simulink model "BLDCmotor_FOC_R2017b_fixdt"  (R2025a)
settings: Solver=FixedStepDiscrete  StartTime=0  StopTime=0.5  FixedStep=Ts  MaxStep=1e-6  RelTol=1e-6  AbsTol=1e-6  EnableMultiTasking=on
PreLoadFcn:
  | addpath(pwd);
  | addpath(genpath('01_Libraries'));
  | addpath(genpath('02_Figures'));
  | addpath(genpath('03_CreateParamTable'));
InitFcn:
  | init_model;
values from neighbouring files (symbols this model uses):
  a_cpr = 65535    [init_model.m]
  a_elecAngle = 60    [init_model.m]
  a_elecoffset = a_elecPeriod/12    (= 30)    [init_model.m]
  a_elecPeriod = 360    [init_model.m]
  a_fcpr = 1/65535    (= 1.52590218967e-05)    [init_model.m]
  a_mechoffset = a_elecoffset/n_polePairs    (= 5)    [init_model.m]
  a_phaAdvMax = 25    [init_model.m]
  b_angleMeasEna = 1    [init_model.m]
  b_cruiseCtrlEna = 0    [init_model.m]
  b_diagEna = 0    [init_model.m]
  b_fieldWeakEna = 0    [init_model.m]
  cf_currFilt = 0.692    [init_model.m]
  cf_idKi = Ki / (f_ctrl)    (= 0.00409061543436)    [init_model.m]
  cf_idKp = Kp    (= 0.0523598775598)    [init_model.m]
  cf_iqKi = Ki / (f_ctrl)    (= 0.00409061543436)    [init_model.m]
  cf_iqKiLimProt = 60 / (f_ctrl)    (= 0.00375)    [init_model.m]
  cf_iqKp = Kp    (= 0.0523598775598)    [init_model.m]
  cf_KbLimProt = Simulink.Parameter    [init_model.m]
  cf_nKi = 20.4 / (f_ctrl)    (= 0.001275)    [init_model.m]
  cf_nKiLimProt = 20 / (f_ctrl)    (= 0.00125)    [init_model.m]
  cf_nKp = 1.18    [init_model.m]
  cf_speedCoef = round(f_ctrl * a_mechAngle * (pi/180) * (30/pi))    [init_model.m]
  CTRL_FOC = 2    [init_model.m]
  CTRL_SIN = 1    [init_model.m]
  dV_openRate = 1000 / (f_ctrl)    (= 0.0625)    [init_model.m]
  dz_cntTrnsDetHi = 40    [init_model.m]
  dz_cntTrnsDetLo = 20    [init_model.m]
  ff_gain = ((r_motn / i_sca) * ((GD32_Vd_max_margin) / v_bus))    (= 0.338958333333)    [init_model.m]
  GD32_Vd_max_margin = GD32_Vd_max - V_margin    (= 1627)    [init_model.m]
  GD32_Vq_max_M1 = sqrt(GD32_Vd_max_margin^2 - GD32_Vq_max_XA.^2)    [init_model.m]
  i_max = i_max * i_sca    (= 500)    [init_model.m]
  id_fieldWeakMax = 5 * i_sca    (= 250)    [init_model.m]
  iq_maxSca_M1 = sqrt(1 - iq_maxSca_XA.^2)    [init_model.m]
  mcu_model = GD32F103    (= 1)    [init_model.m]
  n_commAcvLo = 15    [init_model.m]
  n_commDeacvHi = 30    [init_model.m]
  n_cruiseMotTgt = 0    [init_model.m]
  n_fieldWeakAuthHi = 300    [init_model.m]
  n_fieldWeakAuthLo = 100    [init_model.m]
  n_max = 1950    [init_model.m]
  n_polePairs = 6    [init_model.m]
  n_stdStillDet = 3    [init_model.m]
  OPEN_MODE = 0    [init_model.m]
  r_cos_M1 = cos((a_elecAngle_XA + a_elecPeriod/12)*(pi/180))    [init_model.m]
  r_errInpTgtThres = 600    [init_model.m]
  r_fieldWeakHi = 1000    [init_model.m]
  r_fieldWeakLo = 750    [init_model.m]
  r_motn = r_mot/2    (= 0.25)    [init_model.m]
  r_sin3PhaA_M1 = sin3Arm + A*r_sinPhaA_M1    [init_model.m]
  r_sin3PhaB_M1 = sin3Arm + A*r_sinPhaB_M1    [init_model.m]
  r_sin3PhaC_M1 = sin3Arm + A*r_sinPhaC_M1    [init_model.m]
  r_sin_M1 = sin((a_elecAngle_XA + a_elecPeriod/12)*(pi/180))    [init_model.m]
  SPD_MODE = 2    [init_model.m]
  STM32_Vd_max_margin = STM32_Vd_max - V_margin    (= 940)    [init_model.m]
  STM32_Vq_max_M1 = sqrt(STM32_Vd_max_margin^2 - STM32_Vq_max_XA.^2)    [init_model.m]
  t_errDequal = 1.80 * f_ctrl    (= 28800)    [init_model.m]
  t_errQual = 0.24 * f_ctrl    (= 3840)    [init_model.m]
  tgt_scale = 2047    [init_model.m]
  TRQ_MODE = 3    [init_model.m]
  Ts = 5e-6    (= 5e-06)    [init_model.m]
  Ts_ctrl = 6e-5    (= 6e-05)    [init_model.m]
  v_bus = 24    [init_model.m]
  vec_hallToPos = [0 2 0 1 4 3 5 0]    [init_model.m]
  VLT_MODE = 1    [init_model.m]
  z_commutMap_M1 = [-1 -1  0  1  1  0 ... (first row only)    [init_model.m]
  z_ctrlModReq = TRQ_MODE    (= 3)    [init_model.m]
  z_ctrlTypSel = CTRL_FOC    (= 2)    [init_model.m]
  z_maxCntRst = 2000    [init_model.m]
  z_selPhaCurMeasABC = 2    [init_model.m]
undefined symbols (not defined in the file or in its folder): BLDCmotor_FOC_R2017b_fixdt, DiscIntNeverNeededParam, DWORK0, DWORK1, DWORK2, DWORK3, powergui, spspowerguiLib
libraries: BLDC_controller_Lib x18, simulink x13, prociolib x6, eePwmGenerator x6, eePwmGeneratorMultilevel x3, mcbpositiondecoderlib x2, slpidlib x2, spsControlledVoltageSourceLib x1, spsMultimeterLib x1, spsPermanentMagnetSynchronousMachineLib x1, spsUniversalBridgeLib x1, spsVoltageMeasurementLib x1
(part 4 of 6)

== system BLDCmotor_FOC_R2017b_fixdt/BLDC_controller/F05_Field_Oriented_Control/Clarke_Park_Transform_Forward ==
  note: Start filtering only when motor is enabled (circuit closed).
  b_motEna : Inport
  a_elecAngle : Inport  Port=2
  i_phaAB : Inport  Port=3
  i_phaBC : Inport  Port=4
  Action Port : ActionPort  ActionPortLabel=if(u1 == CTRL_FOC)
  Clarke_Transform : Subsystem
  Current_Filtering : Subsystem
  If2 : If  IfExpression=u1 ~= 0  ShowElse=off
  Park_Transform : Subsystem
  Scope : Scope  NumInputPorts=8
      settings: ActiveDisplayYMinimum=-1177.3322840678534  ActiveDisplayYMaximum=1058.8681928463843  DataLoggingVariableName=ScopeData4
  Sine_Cosine_Approximation : Subsystem
  r_sin : Outport  OutputWhenDisabled=reset  InitialOutput=0  VectorParamsAs1DForOutWhenUnconnected=off
  r_cos : Outport  Port=2  OutputWhenDisabled=reset  InitialOutput=0  VectorParamsAs1DForOutWhenUnconnected=off
  iq : Outport  Port=3  OutputWhenDisabled=reset  InitialOutput=0  VectorParamsAs1DForOutWhenUnconnected=off
  id : Outport  Port=4  OutputWhenDisabled=reset  InitialOutput=0  VectorParamsAs1DForOutWhenUnconnected=off
  iqAbs : Outport  Port=5  OutputWhenDisabled=reset  InitialOutput=0  VectorParamsAs1DForOutWhenUnconnected=off
  wires:
  [a_elecAngle] -> Sine_Cosine_Approximation/1(a_elecAngle)
  Sine_Cosine_Approximation/1(r_sin) -> [r_sin]
  Sine_Cosine_Approximation/2(r_cos) -> [r_cos]
  [b_motEna] -> If2/1
  If2/1 -> Current_Filtering/Action
  Current_Filtering/2(iqAbs) -> [iqAbs]
  [i_phaAB] -> Clarke_Transform/1(i_phaAB)
  [i_phaBC] -> Clarke_Transform/2(i_phaBC)
  Current_Filtering/3(id) -> Scope/4, [id]
  Park_Transform/1(iq_Raw) -> Scope/2, Current_Filtering/1(iq_raw)
  Current_Filtering/1(iq) -> Scope/1, [iq]
  Park_Transform/2(id_Raw) -> Scope/3, Current_Filtering/2(id_raw)
  Clarke_Transform/2(i_beta) -> Scope/6, Park_Transform/2(i_beta)
  [r_cos] -> Scope/8, Park_Transform/4(r_cos)
  [r_sin] -> Scope/7, Park_Transform/3(r_sin)
  Clarke_Transform/1(i_alpha) -> Scope/5, Park_Transform/1(i_apha)
  b_motEna/1 -> [b_motEna]
  i_phaAB/1 -> [i_phaAB]
  i_phaBC/1 -> [i_phaBC]
  a_elecAngle/1 -> [a_elecAngle]
  [id] -> id/1
  [iq] -> iq/1
  [iqAbs] -> iqAbs/1
  [r_cos] -> r_cos/1
  [r_sin] -> r_sin/1

== system BLDCmotor_FOC_R2017b_fixdt/BLDC_controller/F05_Field_Oriented_Control/Clarke_Park_Transform_Inverse ==
  Vq : Inport
  Vd : Inport  Port=2
  r_sin : Inport  Port=3
  r_cos : Inport  Port=4
  Action Port : ActionPort  ActionPortLabel=if(u1 == CTRL_FOC)
  Inv_Clarke_Transform : Subsystem
  Inv_Park_Transform : Subsystem
  Scope : Scope  NumInputPorts=5
      settings: ActiveDisplayYMinimum=-2289.157291869059  ActiveDisplayYMaximum=2435.0032996145992  DataLoggingVariableName=ScopeData3
  V_phaABC_FOC : Outport  OutputWhenDisabled=reset  InitialOutput=0  VectorParamsAs1DForOutWhenUnconnected=off
  wires:
  [V_phaABC_FOC] -> V_phaABC_FOC/1
  Vd/1 -> [Vd]
  r_cos/1 -> [r_cos]
  r_sin/1 -> [r_sin]
  Vq/1 -> [Vq]
  Inv_Clarke_Transform/1(V_phaABC_FOC) -> Scope/5, [V_phaABC_FOC]
  [r_cos] -> Inv_Park_Transform/4(r_cos)
  [Vq] -> Scope/3, Inv_Park_Transform/1(Vq)
  Inv_Park_Transform/1(V_alpha) -> Scope/1, Inv_Clarke_Transform/1(V_alpha)
  Inv_Park_Transform/2(V_beta) -> Scope/4, Inv_Clarke_Transform/2(V_beta)
  [r_sin] -> Inv_Park_Transform/3(r_sin)
  [Vd] -> Scope/2, Inv_Park_Transform/2(Vd)

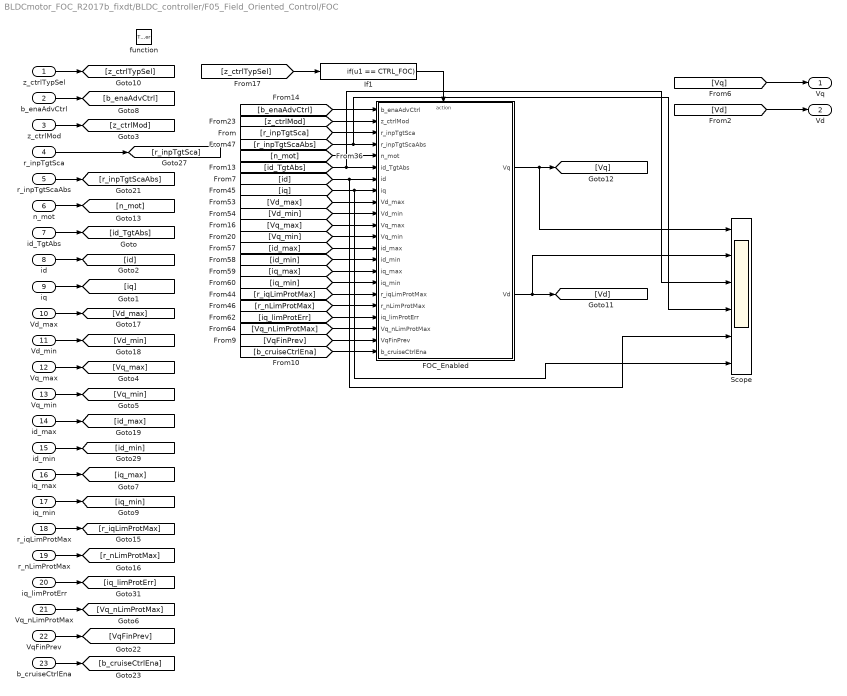
== system BLDCmotor_FOC_R2017b_fixdt/BLDC_controller/F05_Field_Oriented_Control/FOC ==
  z_ctrlTypSel : Inport
  b_enaAdvCtrl : Inport  Port=2
  z_ctrlMod : Inport  Port=3
  r_inpTgtSca : Inport  Port=4
  r_inpTgtScaAbs : Inport  Port=5
  n_mot : Inport  Port=6
  id_TgtAbs : Inport  Port=7
  id : Inport  Port=8
  iq : Inport  Port=9
  Vd_max : Inport  Port=10
  Vd_min : Inport  Port=11
  Vq_max : Inport  Port=12
  Vq_min : Inport  Port=13
  id_max : Inport  Port=14
  id_min : Inport  Port=15
  iq_max : Inport  Port=16
  iq_min : Inport  Port=17
  r_iqLimProtMax : Inport  Port=18
  r_nLimProtMax : Inport  Port=19
  iq_limProtErr : Inport  Port=20
  Vq_nLimProtMax : Inport  Port=21
  VqFinPrev : Inport  Port=22
  b_cruiseCtrlEna : Inport  Port=23
  function : TriggerPort  TriggerType=function-call  VariantControl=Variant
  FOC_Enabled : Subsystem
  If1 : If  IfExpression=u1 == CTRL_FOC  ShowElse=off
  Scope : Scope  NumInputPorts=6
      settings: ActiveDisplayYMinimum=-3867.0934008019167  ActiveDisplayYMaximum=2204.1532756193237  DataLoggingVariableName=ScopeData7
  Vq : Outport  VectorParamsAs1DForOutWhenUnconnected=off
  Vd : Outport  Port=2  VectorParamsAs1DForOutWhenUnconnected=off
  wires:
  [Vq] -> Vq/1
  [Vd] -> Vd/1
  r_inpTgtSca/1 -> [r_inpTgtSca]
  z_ctrlMod/1 -> [z_ctrlMod]
  b_enaAdvCtrl/1 -> [b_enaAdvCtrl]
  iq/1 -> [iq]
  id_min/1 -> [id_min]
  id_max/1 -> [id_max]
  Vd_max/1 -> [Vd_max]
  id_TgtAbs/1 -> [id_TgtAbs]
  id/1 -> [id]
  Vd_min/1 -> [Vd_min]
  Vq_min/1 -> [Vq_min]
  Vq_max/1 -> [Vq_max]
  Vq_nLimProtMax/1 -> [Vq_nLimProtMax]
  iq_limProtErr/1 -> [iq_limProtErr]
  iq_min/1 -> [iq_min]
  iq_max/1 -> [iq_max]
  n_mot/1 -> [n_mot]
  r_iqLimProtMax/1 -> [r_iqLimProtMax]
  r_nLimProtMax/1 -> [r_nLimProtMax]
  r_inpTgtScaAbs/1 -> [r_inpTgtScaAbs]
  VqFinPrev/1 -> [VqFinPrev]
  b_cruiseCtrlEna/1 -> [b_cruiseCtrlEna]
  [b_cruiseCtrlEna] -> FOC_Enabled/22(b_cruiseCtrlEna)
  [r_nLimProtMax] -> FOC_Enabled/18(r_nLimProtMax)
  [r_inpTgtSca] -> FOC_Enabled/3(r_inpTgtSca)
  [r_inpTgtScaAbs] -> Scope/4, FOC_Enabled/4(r_inpTgtScaAbs)
  [Vd_max] -> FOC_Enabled/9(Vd_max)
  [b_enaAdvCtrl] -> FOC_Enabled/1(b_enaAdvCtrl)
  [r_iqLimProtMax] -> FOC_Enabled/17(r_iqLimProtMax)
  [iq_min] -> FOC_Enabled/16(iq_min)
  [iq] -> Scope/6, FOC_Enabled/8(iq)
  [z_ctrlMod] -> FOC_Enabled/2(z_ctrlMod)
  [n_mot] -> FOC_Enabled/5(n_mot)
  [Vq_min] -> FOC_Enabled/12(Vq_min)
  [Vq_nLimProtMax] -> FOC_Enabled/20(Vq_nLimProtMax)
  [id_TgtAbs] -> Scope/3, FOC_Enabled/6(id_TgtAbs)
  [id_max] -> FOC_Enabled/13(id_max)
  [iq_max] -> FOC_Enabled/15(iq_max)
  [Vd_min] -> FOC_Enabled/10(Vd_min)
  [id] -> Scope/5, FOC_Enabled/7(id)
  [VqFinPrev] -> FOC_Enabled/21(VqFinPrev)
  [id_min] -> FOC_Enabled/14(id_min)
  [Vq_max] -> FOC_Enabled/11(Vq_max)
  [iq_limProtErr] -> FOC_Enabled/19(iq_limProtErr)
  [z_ctrlTypSel] -> If1/1
  If1/1 -> FOC_Enabled/Action
  z_ctrlTypSel/1 -> [z_ctrlTypSel]
  FOC_Enabled/1(Vq) -> Scope/1, [Vq]
  FOC_Enabled/2(Vd) -> Scope/2, [Vd]

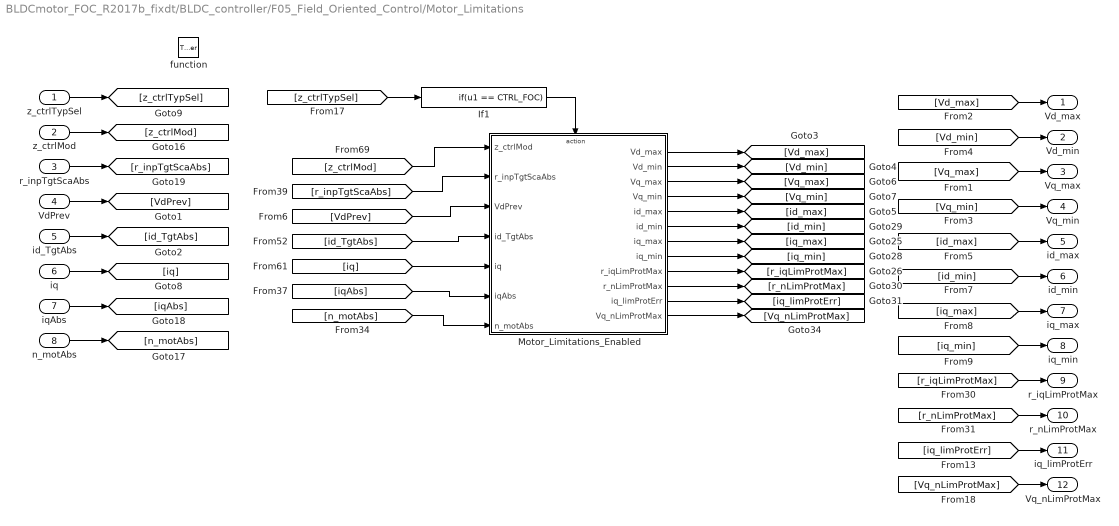
== system BLDCmotor_FOC_R2017b_fixdt/BLDC_controller/F05_Field_Oriented_Control/Motor_Limitations ==
  z_ctrlTypSel : Inport
  z_ctrlMod : Inport  Port=2
  r_inpTgtScaAbs : Inport  Port=3
  VdPrev : Inport  Port=4
  id_TgtAbs : Inport  Port=5
  iq : Inport  Port=6
  iqAbs : Inport  Port=7
  n_motAbs : Inport  Port=8
  function : TriggerPort  TriggerType=function-call  VariantControl=Variant
  If1 : If  IfExpression=u1 == CTRL_FOC  ShowElse=off
  Motor_Limitations_Enabled : Subsystem
  Vd_max : Outport  VectorParamsAs1DForOutWhenUnconnected=off
  Vd_min : Outport  Port=2  VectorParamsAs1DForOutWhenUnconnected=off
  Vq_max : Outport  Port=3  VectorParamsAs1DForOutWhenUnconnected=off
  Vq_min : Outport  Port=4  VectorParamsAs1DForOutWhenUnconnected=off
  id_max : Outport  Port=5  VectorParamsAs1DForOutWhenUnconnected=off
  id_min : Outport  Port=6  VectorParamsAs1DForOutWhenUnconnected=off
  iq_max : Outport  Port=7  VectorParamsAs1DForOutWhenUnconnected=off
  iq_min : Outport  Port=8  VectorParamsAs1DForOutWhenUnconnected=off
  r_iqLimProtMax : Outport  Port=9  VectorParamsAs1DForOutWhenUnconnected=off
  r_nLimProtMax : Outport  Port=10  VectorParamsAs1DForOutWhenUnconnected=off
  iq_limProtErr : Outport  Port=11  VectorParamsAs1DForOutWhenUnconnected=off
  Vq_nLimProtMax : Outport  Port=12  VectorParamsAs1DForOutWhenUnconnected=off
  wires:
  [Vq_min] -> Vq_min/1
  [Vq_max] -> Vq_max/1
  VdPrev/1 -> [VdPrev]
  id_TgtAbs/1 -> [id_TgtAbs]
  [Vd_max] -> Vd_max/1
  [Vd_min] -> Vd_min/1
  [id_min] -> id_min/1
  [id_max] -> id_max/1
  [iq_max] -> iq_max/1
  [iq_min] -> iq_min/1
  iq/1 -> [iq]
  [iq_limProtErr] -> iq_limProtErr/1
  [Vq_nLimProtMax] -> Vq_nLimProtMax/1
  z_ctrlMod/1 -> [z_ctrlMod]
  n_motAbs/1 -> [n_motAbs]
  iqAbs/1 -> [iqAbs]
  r_inpTgtScaAbs/1 -> [r_inpTgtScaAbs]
  [r_nLimProtMax] -> r_nLimProtMax/1
  [r_iqLimProtMax] -> r_iqLimProtMax/1
  [z_ctrlMod] -> Motor_Limitations_Enabled/1(z_ctrlMod)
  [r_inpTgtScaAbs] -> Motor_Limitations_Enabled/2(r_inpTgtScaAbs)
  [VdPrev] -> Motor_Limitations_Enabled/3(VdPrev)
  [id_TgtAbs] -> Motor_Limitations_Enabled/4(id_TgtAbs)
  [iq] -> Motor_Limitations_Enabled/5(iq)
  [iqAbs] -> Motor_Limitations_Enabled/6(iqAbs)
  [n_motAbs] -> Motor_Limitations_Enabled/7(n_motAbs)
  Motor_Limitations_Enabled/1(Vd_max) -> [Vd_max]
  Motor_Limitations_Enabled/2(Vd_min) -> [Vd_min]
  Motor_Limitations_Enabled/3(Vq_max) -> [Vq_max]
  Motor_Limitations_Enabled/4(Vq_min) -> [Vq_min]
  Motor_Limitations_Enabled/5(id_max) -> [id_max]
  Motor_Limitations_Enabled/6(id_min) -> [id_min]
  Motor_Limitations_Enabled/7(iq_max) -> [iq_max]
  Motor_Limitations_Enabled/8(iq_min) -> [iq_min]
  Motor_Limitations_Enabled/9(r_iqLimProtMax) -> [r_iqLimProtMax]
  Motor_Limitations_Enabled/10(r_nLimProtMax) -> [r_nLimProtMax]
  Motor_Limitations_Enabled/11(iq_limProtErr) -> [iq_limProtErr]
  Motor_Limitations_Enabled/12(Vq_nLimProtMax) -> [Vq_nLimProtMax]
  [z_ctrlTypSel] -> If1/1
  If1/1 -> Motor_Limitations_Enabled/Action
  z_ctrlTypSel/1 -> [z_ctrlTypSel]

== system BLDCmotor_FOC_R2017b_fixdt/BLDC_controller/F06_Control_Type_Management/COM_Method ==
  VqFin : Inport
  z_pos : Inport  Port=2
  Action Port : ActionPort  ActionPortLabel=else
  Divide2 : Product  Inputs=**  RndMeth=Simplest  OutDataTypeStr=Inherit: Same as first input
  z_commutMap_M1 : LookupNDDirect  InputsSelectThisObjectFromTable=Vector  Table=z_commutMap_M1  DiagnosticForOutOfRangeInput=None  TableDataTypeStr=int8
  V_phaABC_COM : Outport  VectorParamsAs1DForOutWhenUnconnected=off
  wires:
  Divide2/1 -> [V_phaABC_COM]
  [z_pos] -> z_commutMap_M1/1
  z_commutMap_M1/1 -> Divide2/2
  [VqFin] -> Divide2/1
  VqFin/1 -> [VqFin]
  z_pos/1 -> [z_pos]
  [V_phaABC_COM] -> V_phaABC_COM/1

== system BLDCmotor_FOC_R2017b_fixdt/BLDC_controller/F06_Control_Type_Management/FOC_Method ==
  V_phaABC_FOC_in : Inport
  Action Port : ActionPort  ActionPortLabel=if(u1 ~= 0)
  V_phaABC_FOC : Outport  VectorParamsAs1DForOutWhenUnconnected=off
  wires:
  V_phaABC_FOC_in/1 -> V_phaABC_FOC/1

== system BLDCmotor_FOC_R2017b_fixdt/BLDC_controller/F06_Control_Type_Management/SIN_Method ==
  note: Sinusoidal With 3rd Harmonic
  VqFin : Inport
  a_elecAngle : Inport  Port=2
  z_dir : Inport  Port=3
  r_fieldWeak : Inport  Port=4
  Action Port : ActionPort  ActionPortLabel=elseif(u2 ~= 0)
  Constant : Constant  Value=0  OutDataTypeStr=uint8
  Divide2 : Product  Inputs=**  RndMeth=Simplest  OutDataTypeStr=Inherit: Same as first input
  Final_Phase_Advance_Calculation : Subsystem
  Mux2 : Mux  Inputs=3
  a_elecAngle_XA : PreLookup  BreakpointsData=a_elecAngle_XA  OutputSelection=Index only  IndexSearchMethod=Evenly spaced points  BeginIndexSearchUsingPreviousIndexResult=on  IndexDataTypeStr=uint8  RndMeth=Simplest
  r_sin3PhaA_M1 : Interpolation_n-D  NumberOfTableDimensions=1  Table=r_sin3PhaA_M1  InterpMethod=Flat  ExtrapMethod=Clip  RemoveProtectionIndex=on  ValidIndexMayReachLast=on  OutDataTypeStr=fixdt(1,16,14)  InternalRulePriority=Speed  RndMeth=Simplest
      settings: InputPortMap=u0,u1
  r_sin3PhaB_M1 : Interpolation_n-D  NumberOfTableDimensions=1  Table=r_sin3PhaB_M1  InterpMethod=Flat  ExtrapMethod=Clip  RemoveProtectionIndex=on  ValidIndexMayReachLast=on  OutDataTypeStr=fixdt(1,16,14)  InternalRulePriority=Speed  RndMeth=Simplest
      settings: InputPortMap=u0,u1
  r_sin3PhaC_M1 : Interpolation_n-D  NumberOfTableDimensions=1  Table=r_sin3PhaC_M1  InterpMethod=Flat  ExtrapMethod=Clip  RemoveProtectionIndex=on  ValidIndexMayReachLast=on  OutDataTypeStr=fixdt(1,16,14)  InternalRulePriority=Speed  RndMeth=Simplest
      settings: InputPortMap=u0,u1
  V_phaABC_SIN : Outport  VectorParamsAs1DForOutWhenUnconnected=off
  wires:
  a_elecAngle_XA/1 -> r_sin3PhaC_M1/1, r_sin3PhaB_M1/1, r_sin3PhaA_M1/1
  Constant/1 -> r_sin3PhaC_M1/2, r_sin3PhaB_M1/2, r_sin3PhaA_M1/2
  Final_Phase_Advance_Calculation/1(a_elecAngleAdv) -> a_elecAngle_XA/1
  a_elecAngle/1 -> [a_elecAngle]
  r_fieldWeak/1 -> [r_fieldWeak]
  z_dir/1 -> [z_dir]
  VqFin/1 -> [VqFin]
  [a_elecAngle] -> Final_Phase_Advance_Calculation/1(a_elecAngle)
  [z_dir] -> Final_Phase_Advance_Calculation/2(z_dir)
  [r_fieldWeak] -> Final_Phase_Advance_Calculation/3(r_fieldWeak)
  [V_phaABC_SIN] -> V_phaABC_SIN/1
  [VqFin] -> Divide2/1
  r_sin3PhaA_M1/1 -> Mux2/1
  r_sin3PhaB_M1/1 -> Mux2/2
  r_sin3PhaC_M1/1 -> Mux2/3
  Mux2/1 -> Divide2/2
  Divide2/1 -> [V_phaABC_SIN]

== system BLDCmotor_FOC_R2017b_fixdt/BLDC_model_open1/powergui/EquivalentModel1 ==
  Gates : Subsystem
  Sources : Subsystem
  State-Space : S-Function  FunctionName=sfun_spssw_discc  Parameters=S.Ts,S.A, S.B, S.C, S.D, S.x0, S.EnableUseOfTLC,S.SwitchResistance ,S.SwitchType, S.SwitchGateInitialValue, S.OutputsToResetToZero, S.TBEON,S.SaveMatrices,S.BufferSize  SFunctionDeploymentMode=off  EnableBusSupport=off
  Status : Subsystem
  Yout : Subsystem
  wires:
  State-Space/1 -> Yout/1(v,i)
  State-Space/2 -> Status/1(status)
  Sources/1(u) -> State-Space/1
  Gates/1(gates) -> State-Space/2

== system BLDCmotor_FOC_R2017b_fixdt/PWM_gates/MCU_VD_Selector/Default_Control_Type ==
  1 : Inport
  Action Port : ActionPort
  2 : Outport  VectorParamsAs1DForOutWhenUnconnected=off
  wires:
  1/1 -> 2/1

== system BLDCmotor_FOC_R2017b_fixdt/PWM_gates/MCU_VD_Selector/Default_Control_Type1 ==
  1 : Inport
  Action Port : ActionPort
  2 : Outport  VectorParamsAs1DForOutWhenUnconnected=off
  wires:
  1/1 -> 2/1

== system BLDCmotor_FOC_R2017b_fixdt/PWM_gates/PWM_generator1/__InputSSForSFun__ ==
  DC : Inport  SampleTime=Ts
  __UniqueOutportName__1__ : Outport  VectorParamsAs1DForOutWhenUnconnected=off
  wires:
  DC/1 -> __UniqueOutportName__1__/1

== system BLDCmotor_FOC_R2017b_fixdt/PWM_gates/PWM_generator1/__OutputSSForSFun__ ==
  __UniqueInportName__1__ : Inport
  PWM : Outport  VectorParamsAs1DForOutWhenUnconnected=off
  wires:
  __UniqueInportName__1__/1 -> PWM/1

== system BLDCmotor_FOC_R2017b_fixdt/PWM_gates/PWM_generator12/__InputSSForSFun__ ==
  DC : Inport  SampleTime=Ts
  __UniqueOutportName__1__ : Outport  VectorParamsAs1DForOutWhenUnconnected=off
  wires:
  DC/1 -> __UniqueOutportName__1__/1

== system BLDCmotor_FOC_R2017b_fixdt/PWM_gates/PWM_generator12/__OutputSSForSFun__ ==
  __UniqueInportName__1__ : Inport
  PWM : Outport  VectorParamsAs1DForOutWhenUnconnected=off
  wires:
  __UniqueInportName__1__/1 -> PWM/1

== system BLDCmotor_FOC_R2017b_fixdt/PWM_gates/PWM_generator2/__InputSSForSFun__ ==
  DC : Inport  SampleTime=Ts
  __UniqueOutportName__1__ : Outport  VectorParamsAs1DForOutWhenUnconnected=off
  wires:
  DC/1 -> __UniqueOutportName__1__/1

== system BLDCmotor_FOC_R2017b_fixdt/PWM_gates/PWM_generator2/__OutputSSForSFun__ ==
  __UniqueInportName__1__ : Inport
  PWM : Outport  VectorParamsAs1DForOutWhenUnconnected=off
  wires:
  __UniqueInportName__1__/1 -> PWM/1

== system BLDCmotor_FOC_R2017b_fixdt/PWM_gates/PWM_generator3/__InputSSForSFun__ ==
  DC : Inport  SampleTime=Ts
  __UniqueOutportName__1__ : Outport  VectorParamsAs1DForOutWhenUnconnected=off
  wires:
  DC/1 -> __UniqueOutportName__1__/1

== system BLDCmotor_FOC_R2017b_fixdt/PWM_gates/PWM_generator3/__OutputSSForSFun__ ==
  __UniqueInportName__1__ : Inport
  PWM : Outport  VectorParamsAs1DForOutWhenUnconnected=off
  wires:
  __UniqueInportName__1__/1 -> PWM/1

== system BLDCmotor_FOC_R2017b_fixdt/PWM_gates/PWM_generator4/__InputSSForSFun__ ==
  DC : Inport  SampleTime=Ts
  __UniqueOutportName__1__ : Outport  VectorParamsAs1DForOutWhenUnconnected=off
  wires:
  DC/1 -> __UniqueOutportName__1__/1

== system BLDCmotor_FOC_R2017b_fixdt/PWM_gates/PWM_generator4/__OutputSSForSFun__ ==
  __UniqueInportName__1__ : Inport
  PWM : Outport  VectorParamsAs1DForOutWhenUnconnected=off
  wires:
  __UniqueInportName__1__/1 -> PWM/1

== system BLDCmotor_FOC_R2017b_fixdt/PWM_gates/PWM_generator5/__InputSSForSFun__ ==
  DC : Inport  SampleTime=Ts
  __UniqueOutportName__1__ : Outport  VectorParamsAs1DForOutWhenUnconnected=off
  wires:
  DC/1 -> __UniqueOutportName__1__/1

== system BLDCmotor_FOC_R2017b_fixdt/PWM_gates/PWM_generator5/__OutputSSForSFun__ ==
  __UniqueInportName__1__ : Inport
  PWM : Outport  VectorParamsAs1DForOutWhenUnconnected=off
  wires:
  __UniqueInportName__1__/1 -> PWM/1

== system BLDCmotor_FOC_R2017b_fixdt/Power Stage/Variant Subsystem/GD32F103 ==
  Vd_max1 : Constant  Value=GD32_Vd_max_margin  OutDataTypeStr=fixdt(1,16,4)
  Vd_max_margin : Outport
  wires:
  Vd_max1/1 -> Vd_max_margin/1

== system BLDCmotor_FOC_R2017b_fixdt/Power Stage/Variant Subsystem/STM32F103 ==
  Vd_max3 : Constant  Value=STM32_Vd_max_margin  OutDataTypeStr=fixdt(1,16,4)
  Vd_max_margin : Outport
  wires:
  Vd_max3/1 -> Vd_max_margin/1

== system BLDCmotor_FOC_R2017b_fixdt/BLDC_controller/F01_Estimations/F01_04_Speed_Estimation/Raw_Motor_Speed_Estimation ==
  note: Speed calculations:
      | Speed_radps = (f_ctrl_Hz * Mechanical_angle_radps) / z_counter
      | cf_spd_coef = f_ctrl_Hz * Mechanical_angle_deg * pi/180 * 30/pi
      | Speed_radps = cf_spd_coef / z_counter
  note: Counter hold
  note: • In steady state, switch to 4 interval speed calculation for better accuracy.
      | • In transient, switch to 1 interval interval spped calculation for fast detection of the speed change.
  note: This switch is to manage when direction changes. In this case, the counter measures both the time to go and return (so twice the time) within the Hall change. However, the angle to stand-still is not known. As a work around just use the previous motor speed in absolute value.
  note: At stand-still the Hall sensor toggles if the motor is stoped at the edge of Hall change. This switch is to manage this situation and avoid unexpected behavior.
  z_dir : Inport
  z_dirPrev : Inport  Port=2
  z_counterRawPrev : Inport  Port=3
  n_motAbsPrev : Inport  Port=4
  Action Port : ActionPort  ActionPortLabel=if(u1 ~= 0)
  1-D Lookup Table : Lookup_n-D  Commented=on  NumberOfTableDimensions=1  BreakpointsForDimension1=1:8000  IndexSearchMethod=Evenly spaced points  BeginIndexSearchUsingPreviousIndexResult=on  Table=1 ./ (1:8000)  ExtrapMethod=Clip  RemoveProtectionInput=on  UseLastTableValue=on  ApplyFullPrecisionForLinearInterpolation=on  InternalRulePriority=Speed  OutDataTypeStr=fixdt(0,16,15)  RndMeth=Simplest
  Abs2 : Abs  OutDataTypeStr=Inherit: Inherit via back propagation  RndMeth=Zero  SaturateOnIntegerOverflow=off
  Constant4 : Constant  Value=0  OutDataTypeStr=Inherit: Inherit via back propagation
  Divide11 : Product  Inputs=**  RndMeth=Simplest  OutDataTypeStr=Inherit: Same as first input
  Divide13 : Product  Inputs=*/  OutDataTypeStr=fixdt(1,16,4)  RndMeth=Simplest
  Divide14 : Product  Inputs=*/  OutDataTypeStr=Inherit: Inherit via back propagation  RndMeth=Simplest
  From2 : From  Commented=on  GotoTag=cf_speedCoef
  From3 : From  Commented=on  GotoTag=z_counter
  Logical Operator1 : Logic  AllPortsSameDT=off  OutDataTypeStr=boolean
  Product : Product  Commented=on  OutDataTypeStr=int16  RndMeth=Simplest
  Relational Operator4 : RelationalOperator  Operator=~=  OutDataTypeStr=boolean  RndMeth=Simplest  InputSameDT=off
  Sum1 : Sum  Commented=on  Inputs=++++  InputSameDT=on  RndMeth=Simplest  OutDataTypeStr=Inherit: Same as first input
  Sum13 : Sum  Inputs=++++  InputSameDT=on  RndMeth=Simplest  OutDataTypeStr=Inherit: Same as first input
  Sum7 : Sum  Inputs=+-  InputSameDT=on  RndMeth=Simplest  OutDataTypeStr=Inherit: Same as first input
  Switch1 : Switch  Tag=struct('comment',struct('text','','placement',1),'logdata',struct('maxnumvals',inf,'plotchannels',[],'loggingmode',3,'channels',1),'output',struct('variable','','description','','name','$S_$B','width',1,'address','','max',NaN,'min',NaN,'class','default','type','CONTINUOUS','scaling','','lsb',1,'offset',0,'arb',0,'freeze',1,'unit','','autoscalingmode',1,'lowerheadroom',1,'upperheadroom',1,'headroomunit','bit','keepdatatype',1,'checkmin',0,'checkmax',0,'castoutput',0,'show',0),'threshold',struct('variable','','description','','name','$S_$B_threshold','width',1,'address','','max',NaN,'min',NaN,'class','default','type','CONTINUOUS','scaling','','lsb',1,'offset',0,'arb',0,'freeze',1,'unit','','keepdatatype',1,'value','0','scalar',0,'criteria',3),'scalingvalid',0,'date',733087.49614628474,'inheritscaling',0)  Criteria=u2 ~= 0  SaturateOnIntegerOverflow=off
      settings: AttributesFormatString=threshold=%<threshold>\nCriteria : %<Criteria>
  Switch2 : Switch  Tag=struct('comment',struct('text','','placement',1),'logdata',struct('maxnumvals',inf,'plotchannels',[],'loggingmode',3,'channels',1),'output',struct('variable','','description','','name','$S_$B','width',1,'address','','max',NaN,'min',NaN,'class','default','type','CONTINUOUS','scaling','','lsb',1,'offset',0,'arb',0,'freeze',1,'unit','','autoscalingmode',1,'lowerheadroom',1,'upperheadroom',1,'headroomunit','bit','keepdatatype',1,'checkmin',0,'checkmax',0,'castoutput',0,'show',0),'threshold',struct('variable','','description','','name','$S_$B_threshold','width',1,'address','','max',NaN,'min',NaN,'class','default','type','CONTINUOUS','scaling','','lsb',1,'offset',0,'arb',0,'freeze',1,'unit','','keepdatatype',1,'value','0','scalar',0,'criteria',3),'scalingvalid',0,'date',733087.49614628474,'inheritscaling',0)  Criteria=u2 ~= 0  SaturateOnIntegerOverflow=off
      settings: AttributesFormatString=threshold=%<threshold>\nCriteria : %<Criteria>
  Switch3 : Switch  Tag=struct('comment',struct('text','','placement',1),'logdata',struct('maxnumvals',inf,'plotchannels',[],'loggingmode',3,'channels',1),'output',struct('variable','','description','','name','$S_$B','width',1,'address','','max',NaN,'min',NaN,'class','default','type','CONTINUOUS','scaling','','lsb',1,'offset',0,'arb',0,'freeze',1,'unit','','autoscalingmode',1,'lowerheadroom',1,'upperheadroom',1,'headroomunit','bit','keepdatatype',1,'checkmin',0,'checkmax',0,'castoutput',0,'show',0),'threshold',struct('variable','','description','','name','$S_$B_threshold','width',1,'address','','max',NaN,'min',NaN,'class','default','type','CONTINUOUS','scaling','','lsb',1,'offset',0,'arb',0,'freeze',1,'unit','','keepdatatype',1,'value','0','scalar',0,'criteria',3),'scalingvalid',0,'date',733087.49614628474,'inheritscaling',0)  Criteria=u2 ~= 0  SaturateOnIntegerOverflow=off
      settings: AttributesFormatString=threshold=%<threshold>\nCriteria : %<Criteria>
  UnitDelay{1..5} (5 alike) : UnitDelay  SampleTime=-1  HasFrameUpgradeWarning=on
      settings: AttributesFormatString=Ini=%<X0>
  UnitDelay6 : UnitDelay  Commented=on  SampleTime=-1  HasFrameUpgradeWarning=on
      settings: AttributesFormatString=Ini=%<X0>
  UnitDelay7 : UnitDelay  Commented=on  SampleTime=-1  HasFrameUpgradeWarning=on
      settings: AttributesFormatString=Ini=%<X0>
  UnitDelay8 : UnitDelay  Commented=on  SampleTime=-1  HasFrameUpgradeWarning=on
      settings: AttributesFormatString=Ini=%<X0>
  cf_speedCoef : Constant  Value=cf_speedCoef  OutDataTypeStr=fixdt(0,16,0)
  dz_cntTrnsDet : Relay  OnSwitchValue=dz_cntTrnsDetHi  OffSwitchValue=dz_cntTrnsDetLo  OutDataTypeStr=boolean
  g_Ha : Gain  Commented=on  Gain=4  OutDataTypeStr=Inherit: Inherit via back propagation  RndMeth=Zero  ParamDataTypeStr=Inherit: Same as input
  z_counter : Outport  InitialOutput=z_maxCntRst  VectorParamsAs1DForOutWhenUnconnected=off
  dz_trnsDet : Outport  Port=2  VectorParamsAs1DForOutWhenUnconnected=off
  n_motRaw : Outport  Port=3  VectorParamsAs1DForOutWhenUnconnected=off
  wires:
  z_dir/1 -> [z_dir]
  z_dirPrev/1 -> [z_dirPrev]
  z_counterRawPrev/1 -> [z_counterRawPrev]
  [z_dir] -> Divide11/2
  UnitDelay3/1 -> UnitDelay2/1, Sum13/2
  UnitDelay5/1 -> UnitDelay3/1, Sum13/3
  [z_counter] -> UnitDelay5/1, Sum13/4
  Sum13/1 -> Divide13/2
  [z_counter] -> Divide14/2
  [cf_speedCoef] -> Divide14/1
  UnitDelay4/1 -> Sum7/2
  [z_counter] -> UnitDelay4/1, Sum7/1
  Sum7/1 -> Abs2/1
  Abs2/1 -> dz_cntTrnsDet/1
  cf_speedCoef/1 -> [cf_speedCoef]
  UnitDelay2/1 -> Sum13/1
  [z_dir] -> Relational Operator4/1
  [z_dirPrev] -> Relational Operator4/2
  UnitDelay1/1 -> Logical Operator1/2
  Relational Operator4/1 -> UnitDelay1/1, Switch2/2, Logical Operator1/1
  Logical Operator1/1 -> Switch3/2
  Switch2/1 -> Switch3/3
  Constant4/1 -> Switch3/1
  Switch3/1 -> Divide11/1
  n_motAbsPrev/1 -> [n_motAbsPrev]
  [n_motAbsPrev] -> Switch2/1
  [z_counterRawPrev] -> z_counter/1, [z_counter]
  dz_cntTrnsDet/1 -> [dz_trnsDet], dz_trnsDet/1
  Divide11/1 -> n_motRaw/1
  [dz_trnsDet] -> Switch1/2
  Switch1/1 -> Switch2/3
  Divide14/1 -> Switch1/1
  [cf_speedCoef] -> Divide13/1
  Divide13/1 -> Switch1/3
  UnitDelay8/1 -> UnitDelay7/1, Sum1/3
  Sum1/1 -> 1-D Lookup Table/1
  UnitDelay7/1 -> UnitDelay6/1, Sum1/2
  UnitDelay6/1 -> Sum1/1
  From3/1 -> UnitDelay8/1, Sum1/4
  1-D Lookup Table/1 -> Product/2
  From2/1 -> Product/1

== system BLDCmotor_FOC_R2017b_fixdt/BLDC_controller/F03_Control_Mode_Manager/F03_03_Input_Target_Synthesis/Default_Control_Type ==
  r_inpTgtConv : Inport
  Action Port : ActionPort  ActionPortLabel=else
  r_inpTgtScaDft : Outport  VectorParamsAs1DForOutWhenUnconnected=off
  wires:
  r_inpTgtConv/1 -> r_inpTgtScaDft/1

== system BLDCmotor_FOC_R2017b_fixdt/BLDC_controller/F03_Control_Mode_Manager/F03_03_Input_Target_Synthesis/Default_Mode ==
  r_inpTgtScaRaw : Inport
  Action Port : ActionPort  InitializeStates=reset  ActionPortLabel=else
  r_inpTgtScaDft : Outport  VectorParamsAs1DForOutWhenUnconnected=off
  wires:
  r_inpTgtScaRaw/1 -> r_inpTgtScaDft/1

== system BLDCmotor_FOC_R2017b_fixdt/BLDC_controller/F03_Control_Mode_Manager/F03_03_Input_Target_Synthesis/FOC_Control_Type ==
  r_inpTgtConv : Inport
  z_ctrlModReq : Inport  Port=2
  Action Port : ActionPort  ActionPortLabel=if(u1 == CTRL_FOC)
  Divide1 : Product  Inputs=**  RndMeth=Simplest  OutDataTypeStr=Inherit: Same as first input
  Divide4 : Product  Inputs=*/  OutDataTypeStr=fixdt(0,16,14)  RndMeth=Simplest
  Mux : Mux
  Selector : Selector  IndexMode=Zero-based  InputPortWidth=4  IndexOptions=Index vector (port)  Indices=[1 3]  OutputSizes=1
  Variant Subsystem1 : Subsystem  Variant=on  VariantActivationTime=code compile
  constant : Constant  Value=tgt_scale  OutDataTypeStr=Inherit: Inherit via back propagation
  constant1 : Constant  Value=0  OutDataTypeStr=Inherit: Inherit via back propagation
  i_max : Constant  Value=i_max  OutDataTypeStr=fixdt(1,16,4)
  n_max : Constant  Value=n_max  OutDataTypeStr=fixdt(1,16,4)
  r_inpTgtScaFOC : Outport  VectorParamsAs1DForOutWhenUnconnected=off
  wires:
  r_inpTgtConv/1 -> [r_inpTgtConv]
  [r_inpTgtScaFOC] -> r_inpTgtScaFOC/1
  z_ctrlModReq/1 -> [z_ctrlModReq]
  constant/1 -> Divide4/2
  Selector/1 -> Divide4/1
  constant1/1 -> Mux/1
  i_max/1 -> Mux/4
  Mux/1 -> Selector/1
  n_max/1 -> Mux/3
  [z_ctrlModReq] -> Selector/2
  Divide4/1 -> Divide1/2
  Divide1/1 -> [r_inpTgtScaFOC]
  [r_inpTgtConv] -> Divide1/1
  Variant Subsystem1/1(Vd_max_margin) -> Mux/2

== system BLDCmotor_FOC_R2017b_fixdt/BLDC_controller/F03_Control_Mode_Manager/F03_03_Input_Target_Synthesis/Open_Mode ==
  note: In case of OPEN_MODE request the input target command will be reduced to 0 with a predefined rate.
  VqFinPrev : Inport
  Action Port : ActionPort  InitializeStates=reset  ActionPortLabel=if(u1 == OPEN_MODE)
  Constant23 : Constant  Value=0  OutDataTypeStr=Inherit: Inherit via back propagation
  Data Type Conversion : DataTypeConversion  OutDataTypeStr=fixdt(1,28,16)  SaturateOnIntegerOverflow=off  RndMeth=Floor
  Data Type Conversion1 : DataTypeConversion  OutDataTypeStr=fixdt(1,16,4)  SaturateOnIntegerOverflow=off  RndMeth=Floor
  Gain3 : Gain  Tag=struct('comment',struct('text','','placement',1),'logdata',struct('maxnumvals',inf,'plotchannels',[],'loggingmode',3,'channels',1),'output',struct('variable','','description','','name','$S_$B','width',1,'address','','max',NaN,'min',NaN,'class','default','type','CONTINUOUS','scaling','','lsb',1,'offset',0,'arb',0,'freeze',1,'unit','','autoscalingmode',1,'lowerheadroom',1,'upperheadroom',1,'headroomunit','bit','keepdatatype',1,'checkmin',0,'checkmax',0,'castoutput',0,'show',0),'gain',struct('variable','','description','','name','$S_$B_gain','width',1,'address','','max',NaN,'min',NaN,'class','default','type','CONTINUOUS','scaling','','lsb',1,'offset',0,'arb',0,'freeze',1,'unit','','keepdatatype',1,'value','1','scalar',0,'tolerance',1),'scalingvalid',0,'date',730486)  Gain=-1  RndMeth=Zero  OutDataTypeStr=Inherit: Same as input
  Rate_Limiter : BLDC_controller_Lib/Rate_Limiter  SystemSampleTime=-1  VariantActivationTime=update diagram  EmptyChoice=off  PassThrough=off  PassThroughVariantControl=(default)  EmptyChoiceVariantControl=(default)  AllowFlexibleInterface=on  Latency=0  AutoFrameSizeCalculation=off
  dV_openRate : Constant  Value=dV_openRate  OutDataTypeStr=fixdt(1,28,16)
  rising_edge_init : BLDC_controller_Lib/rising_edge_init
  r_inpTgtScaOpen : Outport  VectorParamsAs1DForOutWhenUnconnected=off
  wires:
  VqFinPrev/1 -> [VqFinPrev]
  Constant23/1 -> Rate_Limiter/1
  rising_edge_init/1 -> Rate_Limiter/3
  Gain3/1 -> Rate_Limiter/5
  dV_openRate/1 -> Gain3/1, Rate_Limiter/4
  Data Type Conversion1/1 -> [r_inpTgtScaOpen]
  [r_inpTgtScaOpen] -> r_inpTgtScaOpen/1
  Rate_Limiter/1 -> Data Type Conversion1/1
  [VqFinPrev] -> Data Type Conversion/1
  Data Type Conversion/1 -> Rate_Limiter/2

== system BLDCmotor_FOC_R2017b_fixdt/BLDC_controller/F05_Field_Oriented_Control/Clarke_Park_Transform_Forward/Clarke_Transform ==
  i_phaAB : Inport
  i_phaBC : Inport  Port=2
  Clarke_PhasesAB : Subsystem
  Clarke_PhasesAC : Subsystem
  Clarke_PhasesBC : Subsystem
  If1 : If  IfExpression=u1 == 0  ElseIfExpressions=u1 == 1
  Merge1 : Merge  Inputs=3
  Merge2 : Merge  Inputs=3
  Scope : Scope  NumInputPorts=4
      settings: ActiveDisplayYMinimum=-661.83017116928522  ActiveDisplayYMaximum=246.20015638161976  DataLoggingVariableName=ScopeData8
  z_selPhaCurMeasABC : Constant  Value=z_selPhaCurMeasABC  OutDataTypeStr=uint8
  i_alpha : Outport  VectorParamsAs1DForOutWhenUnconnected=off
  i_beta : Outport  Port=2  VectorParamsAs1DForOutWhenUnconnected=off
  wires:
  Clarke_PhasesBC/1(i_alphaBC) -> [i_alphaBC]
  [i_betaBC] -> Merge1/2
  [i_betaAB] -> Merge1/1
  i_phaAB/1 -> [i_phaAB]
  [i_phaBC] -> Clarke_PhasesBC/2(i_phaC)
  [i_phaAB] -> Clarke_PhasesBC/1(i_phaB)
  Clarke_PhasesAB/1(i_alphaAB) -> [i_alphaAB]
  [i_alphaAB] -> Merge2/1
  If1/1 -> Clarke_PhasesAB/Action
  z_selPhaCurMeasABC/1 -> If1/1
  [i_alphaBC] -> Merge2/2
  [i_beta] -> i_beta/1
  Clarke_PhasesAB/2(i_betaAB) -> [i_betaAB]
  i_phaBC/1 -> [i_phaBC]
  [i_phaBC] -> Scope/2, Clarke_PhasesAB/2(i_phaB)
  Merge2/1 -> Scope/3, [i_alpha]
  [i_phaAB] -> Scope/1, Clarke_PhasesAB/1(i_phaA)
  [i_alpha] -> i_alpha/1
  Clarke_PhasesBC/2(i_betaBC) -> [i_betaBC]
  If1/2 -> Clarke_PhasesBC/Action
  If1/3 -> Clarke_PhasesAC/Action
  [i_phaAB] -> Clarke_PhasesAC/1(i_phaA)
  [i_phaBC] -> Clarke_PhasesAC/2(i_phaC)
  Clarke_PhasesAC/2(i_betaAC) -> [i_betaAC]
  Clarke_PhasesAC/1(i_alphaAC) -> [i_alphaAC]
  [i_alphaAC] -> Merge2/3
  [i_betaAC] -> Merge1/3
  Merge1/1 -> Scope/4, [i_beta]

== system BLDCmotor_FOC_R2017b_fixdt/BLDC_controller/F05_Field_Oriented_Control/Clarke_Park_Transform_Forward/Current_Filtering ==
  iq_raw : Inport
  id_raw : Inport  Port=2
  Action Port : ActionPort  InitializeStates=reset  ActionPortLabel=if(u1 ~= 0)
  Abs5 : Abs  OutDataTypeStr=Inherit: Inherit via back propagation  RndMeth=Zero  SaturateOnIntegerOverflow=off
  Demux1 : Demux  Outputs=2
  Low_Pass_Filter : BLDC_controller_Lib/Low_Pass_Filter  SystemSampleTime=-1  VariantActivationTime=update diagram  EmptyChoice=off  PassThrough=off  PassThroughVariantControl=(default)  EmptyChoiceVariantControl=(default)  AllowFlexibleInterface=on  Latency=0  AutoFrameSizeCalculation=off
  Mux2 : Mux  Inputs=2
  cf_currFilt : Constant  Value=cf_currFilt  OutDataTypeStr=fixdt(0,16,16)
  iq : Outport  OutputWhenDisabled=reset  InitialOutput=0  VectorParamsAs1DForOutWhenUnconnected=off
  iqAbs : Outport  Port=2  OutputWhenDisabled=reset  InitialOutput=0  VectorParamsAs1DForOutWhenUnconnected=off
  id : Outport  Port=3  OutputWhenDisabled=reset  InitialOutput=0  VectorParamsAs1DForOutWhenUnconnected=off
  wires:
  Mux2/1 -> Low_Pass_Filter/1
  Demux1/2 -> [id]
  cf_currFilt/1 -> Low_Pass_Filter/2
  id_raw/1 -> [id_raw]
  [iq] -> iq/1, Abs5/1
  [id] -> id/1
  iq_raw/1 -> [iq_raw]
  Demux1/1 -> [iq]
  Low_Pass_Filter/1 -> Demux1/1
  [iq_raw] -> Mux2/1
  [id_raw] -> Mux2/2
  Abs5/1 -> iqAbs/1

== system BLDCmotor_FOC_R2017b_fixdt/BLDC_controller/F05_Field_Oriented_Control/Clarke_Park_Transform_Forward/Park_Transform ==
  note: Park Transform:
      | iq = -i_alpha*sin(angle) + i_beta*cos(angle)
      | id = i_alpha*cos(angle) + i_beta*sin(angle)
  i_apha : Inport
  i_beta : Inport  Port=2
  r_sin : Inport  Port=3
  r_cos : Inport  Port=4
  Divide{1..4} (4 alike) : Product  Inputs=**  RndMeth=Simplest  OutDataTypeStr=Inherit: Same as first input
  Sum1 : Sum  OutDataTypeStr=Inherit: Inherit via back propagation  RndMeth=Simplest  SaturateOnIntegerOverflow=on
  Sum6 : Sum  Inputs=-+  OutDataTypeStr=Inherit: Inherit via back propagation  RndMeth=Simplest  SaturateOnIntegerOverflow=on
  iq_Raw : Outport  VectorParamsAs1DForOutWhenUnconnected=off
  id_Raw : Outport  Port=2  VectorParamsAs1DForOutWhenUnconnected=off
  wires:
  r_sin/1 -> [r_sin]
  i_beta/1 -> [i_beta]
  i_apha/1 -> [i_apha]
  r_cos/1 -> [r_cos]
  [r_sin] -> Divide4/2
  [i_apha] -> Divide4/1
  Divide4/1 -> Sum6/1
  Divide1/1 -> Sum6/2
  [i_beta] -> Divide1/1
  [r_cos] -> Divide1/2
  Sum6/1 -> iq_Raw/1
  Divide2/1 -> Sum1/1
  [i_apha] -> Divide2/1
  [r_cos] -> Divide2/2
  Divide3/1 -> Sum1/2
  [i_beta] -> Divide3/1
  [r_sin] -> Divide3/2
  Sum1/1 -> id_Raw/1

== system BLDCmotor_FOC_R2017b_fixdt/BLDC_controller/F05_Field_Oriented_Control/Clarke_Park_Transform_Forward/Sine_Cosine_Approximation ==
  note: Sine/Cosine Look-up Tables
  note: Note: The Sine and Cosine maps are shifted in phase by 30 deg to align with the Hall sensors position.
  a_elecAngle : Inport
  a_elecAngle_XA : PreLookup  BreakpointsData=a_elecAngle_XA  OutputSelection=Index and fraction as bus  IndexSearchMethod=Evenly spaced points  BeginIndexSearchUsingPreviousIndexResult=on  UseLastBreakpoint=on  RemoveProtectionInput=on  IndexDataTypeStr=uint8  FractionDataTypeStr=fixdt(0,16,15)  RndMeth=Simplest
  r_cos_M1 : Interpolation_n-D  NumberOfTableDimensions=1  Table=r_cos_M1  ExtrapMethod=Clip  DiagnosticForOutOfRangeInput=Error  RequireIndexFractionAsBus=on  RemoveProtectionIndex=on  ValidIndexMayReachLast=on  OutDataTypeStr=fixdt(1,16,14)  InternalRulePriority=Speed  RndMeth=Simplest
      settings: InputPortMap=u0
  r_sin_M1 : Interpolation_n-D  NumberOfTableDimensions=1  Table=r_sin_M1  ExtrapMethod=Clip  DiagnosticForOutOfRangeInput=Error  RequireIndexFractionAsBus=on  RemoveProtectionIndex=on  ValidIndexMayReachLast=on  OutDataTypeStr=fixdt(1,16,14)  InternalRulePriority=Speed  RndMeth=Simplest
      settings: InputPortMap=u0
  r_sin : Outport  VectorParamsAs1DForOutWhenUnconnected=off
  r_cos : Outport  Port=2  VectorParamsAs1DForOutWhenUnconnected=off
  wires:
  a_elecAngle_XA/1 -> r_cos_M1/1, r_sin_M1/1
  a_elecAngle/1 -> [a_elecAngle]
  [r_sin] -> r_sin/1
  r_sin_M1/1 -> [r_sin]
  [r_cos] -> r_cos/1
  r_cos_M1/1 -> [r_cos]
  [a_elecAngle] -> a_elecAngle_XA/1

== system BLDCmotor_FOC_R2017b_fixdt/BLDC_controller/F05_Field_Oriented_Control/Clarke_Park_Transform_Inverse/Inv_Clarke_Transform ==
  note: Inverse Clarke Transform:
      | V_phaA = V_alpha
      | V_phaB = -(1/2)*V_alpha + (sqrt(3)/2)*V_beta
      | V_phaC = -VphaA - V_phaB
  note: Space Vector Modulation (SVM)
  V_alpha : Inport
  V_beta : Inport  Port=2
  Add : Sum  SaturateOnIntegerOverflow=on
  Add1 : Sum  Inputs=-+  SaturateOnIntegerOverflow=on  OutDataTypeStr=Inherit: Same as first input
  Gain1 : Gain  Tag=struct('comment',struct('text','','placement',1),'logdata',struct('maxnumvals',inf,'plotchannels',[],'loggingmode',3,'channels',1),'output',struct('variable','','description','','name','$S_$B','width',1,'address','','max',NaN,'min',NaN,'class','default','type','CONTINUOUS','scaling','','lsb',1,'offset',0,'arb',0,'freeze',1,'unit','','autoscalingmode',1,'lowerheadroom',1,'upperheadroom',1,'headroomunit','bit','keepdatatype',1,'checkmin',0,'checkmax',0,'castoutput',0,'show',0),'gain',struct('variable','','description','','name','$S_$B_gain','width',1,'address','','max',NaN,'min',NaN,'class','default','type','CONTINUOUS','scaling','','lsb',1,'offset',0,'arb',0,'freeze',1,'unit','','keepdatatype',1,'value','1','scalar',0,'tolerance',1),'scalingvalid',0,'date',730486)  Gain=sqrt(3)/2  RndMeth=Zero  OutDataTypeStr=Inherit: Same as input
  Gain2 : Gain  Gain=0.5  OutDataTypeStr=Inherit: Same as input
  Gain3 : Gain  Tag=struct('comment',struct('text','','placement',1),'logdata',struct('maxnumvals',inf,'plotchannels',[],'loggingmode',3,'channels',1),'output',struct('variable','','description','','name','$S_$B','width',1,'address','','max',NaN,'min',NaN,'class','default','type','CONTINUOUS','scaling','','lsb',1,'offset',0,'arb',0,'freeze',1,'unit','','autoscalingmode',1,'lowerheadroom',1,'upperheadroom',1,'headroomunit','bit','keepdatatype',1,'checkmin',0,'checkmax',0,'castoutput',0,'show',0),'gain',struct('variable','','description','','name','$S_$B_gain','width',1,'address','','max',NaN,'min',NaN,'class','default','type','CONTINUOUS','scaling','','lsb',1,'offset',0,'arb',0,'freeze',1,'unit','','keepdatatype',1,'value','1','scalar',0,'tolerance',1),'scalingvalid',0,'date',730486)  Gain=1/2  RndMeth=Zero  OutDataTypeStr=Inherit: Same as input
  Gain4 : Gain  Gain=2/sqrt(3)  OutDataTypeStr=Inherit: Same as input
  MinMax1 : MinMax  InputSameDT=on
  MinMax2 : MinMax  Function=max  InputSameDT=on
  Mux4 : Mux  Inputs=3
  Sum2 : Sum  Inputs=--  RndMeth=Simplest  SaturateOnIntegerOverflow=on  OutDataTypeStr=Inherit: Same as first input
  Sum6 : Sum  Inputs=-+  RndMeth=Simplest  SaturateOnIntegerOverflow=on  OutDataTypeStr=Inherit: Same as first input
  V_phaABC_FOC : Outport  VectorParamsAs1DForOutWhenUnconnected=off
  wires:
  Sum6/1 -> Sum2/2, Mux4/2
  Sum2/1 -> Mux4/3
  Gain1/1 -> Sum6/2
  Gain3/1 -> Sum6/1
  V_alpha/1 -> Gain3/1, Sum2/1, Mux4/1  "alpha"
  V_beta/1 -> Gain1/1  "beta"
  Add/1 -> Gain2/1
  Add1/1 -> Gain4/1
  MinMax1/1 -> Add/1
  Gain2/1 -> Add1/1
  Gain4/1 -> V_phaABC_FOC/1
  MinMax2/1 -> Add/2
  Mux4/1 -> Add1/2, MinMax2/1, MinMax1/1

== system BLDCmotor_FOC_R2017b_fixdt/BLDC_controller/F05_Field_Oriented_Control/Clarke_Park_Transform_Inverse/Inv_Park_Transform ==
  note: Inverse Park Transform:
      | V_alpha = Vd*cos(angle) - Vq*sin(angle)
      | V_beta = Vd*sin(angle) + Vq*cos(angle)
  Vq : Inport
  Vd : Inport  Port=2
  r_sin : Inport  Port=3
  r_cos : Inport  Port=4
  Divide{1..4} (4 alike) : Product  Inputs=**  RndMeth=Simplest  OutDataTypeStr=Inherit: Same as first input
  Sum1 : Sum  RndMeth=Simplest  SaturateOnIntegerOverflow=on  OutDataTypeStr=Inherit: Same as first input
  Sum6 : Sum  Inputs=+-  RndMeth=Simplest  SaturateOnIntegerOverflow=on  OutDataTypeStr=Inherit: Same as first input
  V_alpha : Outport  VectorParamsAs1DForOutWhenUnconnected=off
  V_beta : Outport  Port=2  VectorParamsAs1DForOutWhenUnconnected=off
  wires:
  r_sin/1 -> [r_sin]
  Vd/1 -> [Vd]
  Vq/1 -> [Vq]
  r_cos/1 -> [r_cos]
  [r_cos] -> Divide4/2
  [r_sin] -> Divide1/2
  [Vd] -> Divide4/1
  [r_cos] -> Divide3/2
  Divide1/1 -> Sum6/2
  [Vq] -> Divide1/1
  [Vd] -> Divide2/1
  Divide2/1 -> Sum1/1
  Divide3/1 -> Sum1/2
  [Vq] -> Divide3/1
  Divide4/1 -> Sum6/1
  [r_sin] -> Divide2/2
  Sum1/1 -> V_beta/1
  Sum6/1 -> V_alpha/1

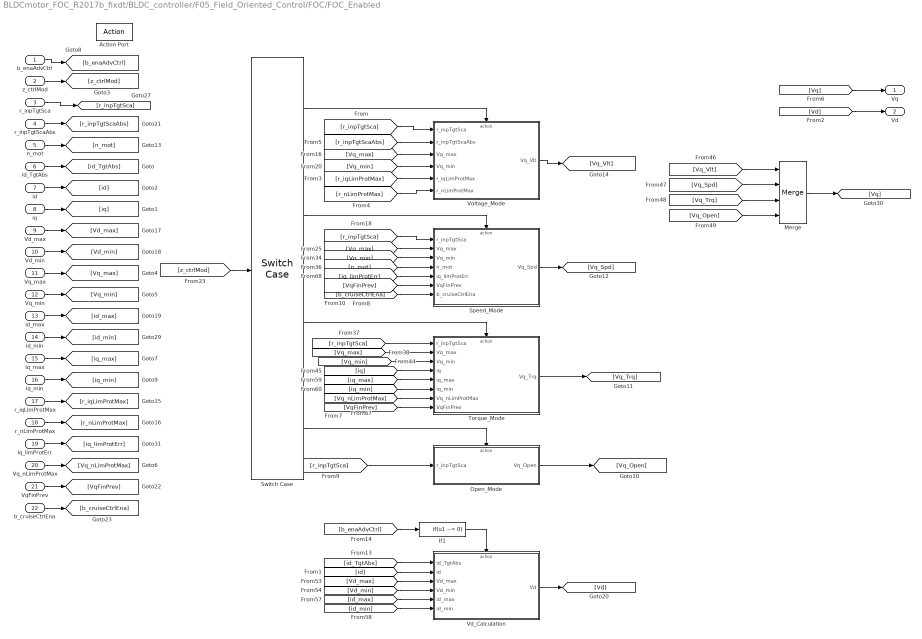
== system BLDCmotor_FOC_R2017b_fixdt/BLDC_controller/F05_Field_Oriented_Control/FOC/FOC_Enabled ==
  b_enaAdvCtrl : Inport
  z_ctrlMod : Inport  Port=2
  r_inpTgtSca : Inport  Port=3
  r_inpTgtScaAbs : Inport  Port=4
  n_mot : Inport  Port=5
  id_TgtAbs : Inport  Port=6
  id : Inport  Port=7
  iq : Inport  Port=8
  Vd_max : Inport  Port=9
  Vd_min : Inport  Port=10
  Vq_max : Inport  Port=11
  Vq_min : Inport  Port=12
  id_max : Inport  Port=13
  id_min : Inport  Port=14
  iq_max : Inport  Port=15
  iq_min : Inport  Port=16
  r_iqLimProtMax : Inport  Port=17
  r_nLimProtMax : Inport  Port=18
  iq_limProtErr : Inport  Port=19
  Vq_nLimProtMax : Inport  Port=20
  VqFinPrev : Inport  Port=21
  b_cruiseCtrlEna : Inport  Port=22
  Action Port : ActionPort  ActionPortLabel=if(u1 == CTRL_FOC)
  If1 : If  IfExpression=u1 ~= 0  ShowElse=off
  Merge : Merge  Inputs=4
  Open_Mode : Subsystem
  Speed_Mode : Subsystem
  Switch Case : SwitchCase  CaseConditions={VLT_MODE, SPD_MODE, TRQ_MODE}
  Torque_Mode : Subsystem
  Vd_Calculation : Subsystem
  Voltage_Mode : Subsystem
  Vq : Outport  VectorParamsAs1DForOutWhenUnconnected=off
  Vd : Outport  Port=2  VectorParamsAs1DForOutWhenUnconnected=off
  wires:
  [id_TgtAbs] -> Vd_Calculation/1(id_TgtAbs)
  [z_ctrlMod] -> Switch Case/1
  If1/1 -> Vd_Calculation/Action
  [id] -> Vd_Calculation/2(id)
  [b_enaAdvCtrl] -> If1/1
  Torque_Mode/1(Vq_Trq) -> [Vq_Trq]
  Switch Case/3 -> Torque_Mode/Action
  [Vq_min] -> Speed_Mode/3(Vq_min)
  [Vq_Vlt] -> Merge/1
  [n_mot] -> Speed_Mode/4(n_mot)
  [Vq_max] -> Speed_Mode/2(Vq_max)
  Switch Case/2 -> Speed_Mode/Action
  [Vq_Open] -> Merge/4
  [r_inpTgtSca] -> Voltage_Mode/1(r_inpTgtSca)
  [r_inpTgtSca] -> Speed_Mode/1(r_inpTgtSca)
  [Vq_max] -> Voltage_Mode/3(Vq_max)
  [Vq_min] -> Voltage_Mode/4(Vq_min)
  Switch Case/1 -> Voltage_Mode/Action
  Switch Case/4 -> Open_Mode/Action
  [Vq_Spd] -> Merge/2
  [Vq_Trq] -> Merge/3
  Speed_Mode/1(Vq_Spd) -> [Vq_Spd]
  Open_Mode/1(Vq_Open) -> [Vq_Open]
  Voltage_Mode/1(Vq_Vlt) -> [Vq_Vlt]
  [Vd_max] -> Vd_Calculation/3(Vd_max)
  [r_inpTgtSca] -> Open_Mode/1(r_inpTgtSca)
  [id_min] -> Vd_Calculation/6(id_min)
  [id_max] -> Vd_Calculation/5(id_max)
  [Vd_min] -> Vd_Calculation/4(Vd_min)
  [iq_limProtErr] -> Speed_Mode/5(iq_limProtErr)
  [Vq] -> Vq/1
  [Vd] -> Vd/1
  r_inpTgtSca/1 -> [r_inpTgtSca]
  z_ctrlMod/1 -> [z_ctrlMod]
  b_enaAdvCtrl/1 -> [b_enaAdvCtrl]
  iq/1 -> [iq]
  id_min/1 -> [id_min]
  id_max/1 -> [id_max]
  Vd_max/1 -> [Vd_max]
  id_TgtAbs/1 -> [id_TgtAbs]
  id/1 -> [id]
  Vd_min/1 -> [Vd_min]
  Vq_min/1 -> [Vq_min]
  Vq_max/1 -> [Vq_max]
  Vq_nLimProtMax/1 -> [Vq_nLimProtMax]
  iq_limProtErr/1 -> [iq_limProtErr]
  iq_min/1 -> [iq_min]
  iq_max/1 -> [iq_max]
  n_mot/1 -> [n_mot]
  r_iqLimProtMax/1 -> [r_iqLimProtMax]
  r_nLimProtMax/1 -> [r_nLimProtMax]
  [r_iqLimProtMax] -> Voltage_Mode/5(r_iqLimProtMax)
  [r_nLimProtMax] -> Voltage_Mode/6(r_nLimProtMax)
  r_inpTgtScaAbs/1 -> [r_inpTgtScaAbs]
  [r_inpTgtScaAbs] -> Voltage_Mode/2(r_inpTgtScaAbs)
  VqFinPrev/1 -> [VqFinPrev]
  [VqFinPrev] -> Speed_Mode/6(VqFinPrev)
  [b_cruiseCtrlEna] -> Speed_Mode/7(b_cruiseCtrlEna)
  b_cruiseCtrlEna/1 -> [b_cruiseCtrlEna]
  Vd_Calculation/1(Vd) -> [Vd]
  Merge/1 -> [Vq]
  [r_inpTgtSca] -> Torque_Mode/1(r_inpTgtSca)
  [Vq_max] -> Torque_Mode/2(Vq_max)
  [Vq_min] -> Torque_Mode/3(Vq_min)
  [iq] -> Torque_Mode/4(iq)
  [iq_max] -> Torque_Mode/5(iq_max)
  [iq_min] -> Torque_Mode/6(iq_min)
  [Vq_nLimProtMax] -> Torque_Mode/7(Vq_nLimProtMax)
  [VqFinPrev] -> Torque_Mode/8(VqFinPrev)
